simulink model "rusticone"  (R2018b)
settings: Solver=VariableStepAuto  StartTime=0.0  StopTime=10.0  RelTol=1e-3
libraries: simulink_extras x1, simulink x1
settings Model: Creator=Edoardo  LastModifiedBy=Edoardo

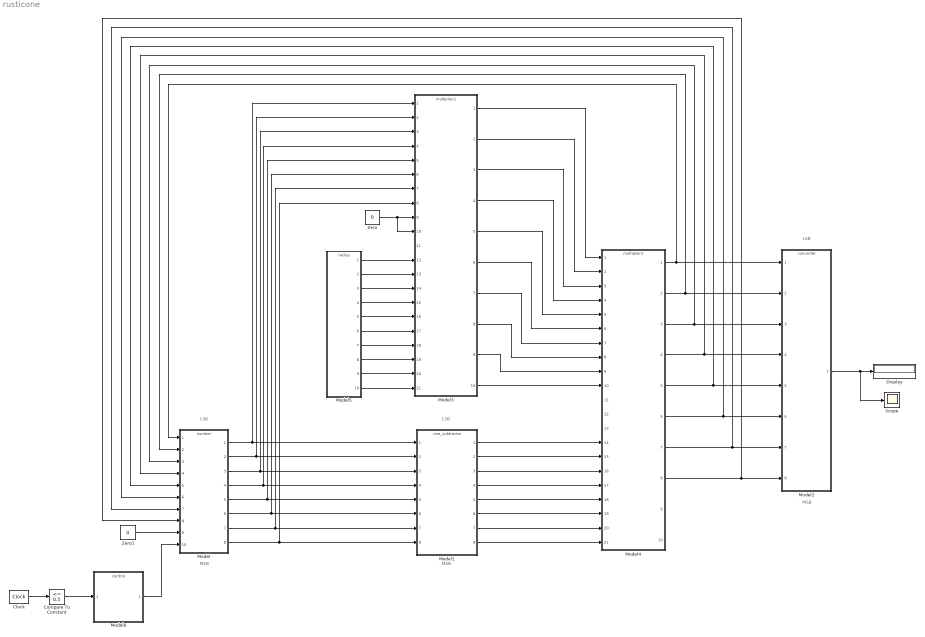
== system rusticone ==
  note: LSB
  note: LSB
  note: MSB
  note: LSB
  note: MSB
  note: MSB
  Clock : simulink_extras/Flip Flops/Clock  period=2
  Compare To Constant : simulink/Logic and Bit Operations/Compare To Constant  relop=<=  const=0.5  OutDataTypeStr=boolean  ZeroCross=off
  Display : Display
  Model : ModelReference  ModelNameDialog=number  SimulationMode=Normal  ModelReferenceVersion=1.14
  Model1 : ModelReference  ModelNameDialog=one_subtractor  SimulationMode=Normal  ModelReferenceVersion=1.7
  Model2 : ModelReference  ModelNameDialog=converter  SimulationMode=Normal  ModelReferenceVersion=1.8
  Model3 : ModelReference  ModelNameDialog=multiplier2.slx  SimulationMode=Normal  ModelReferenceVersion=1.12
  Model4 : ModelReference  ModelNameDialog=multiplier2.slx  SimulationMode=Normal  ModelReferenceVersion=1.12
  Model5 : ModelReference  ModelNameDialog=radius  SimulationMode=Normal  ModelReferenceVersion=1.3
  Model6 : ModelReference  ModelNameDialog=control  SimulationMode=Normal  ModelReferenceVersion=1.1
  Scope : Scope
  Zero : Constant  Value=0  OutDataTypeStr=Inherit: Inherit via back propagation
  Zero1 : Constant  Value=0  OutDataTypeStr=Inherit: Inherit via back propagation
  wires:
  Model2/1 -> Scope/1, Display/1
  Model/1 -> Model3/1, Model1/1
  Model/6 -> Model3/6, Model1/6
  Model/7 -> Model3/7, Model1/7
  Model/4 -> Model1/4, Model3/4
  Model/8 -> Model3/8, Model1/8
  Model/2 -> Model3/2, Model1/2
  Model/5 -> Model3/5, Model1/5
  Model/3 -> Model3/3, Model1/3
  Model3/1 -> Model4/1
  Model3/2 -> Model4/2
  Model3/3 -> Model4/3
  Model3/4 -> Model4/4
  Model3/5 -> Model4/5
  Model3/6 -> Model4/6
  Model3/7 -> Model4/7
  Model3/8 -> Model4/8
  Model3/9 -> Model4/9
  Model3/10 -> Model4/10
  Model1/1 -> Model4/14
  Model1/2 -> Model4/15
  Model1/3 -> Model4/16
  Model1/4 -> Model4/17
  Model1/5 -> Model4/18
  Model1/6 -> Model4/19
  Model1/7 -> Model4/20
  Model1/8 -> Model4/21
  Zero/1 -> Model3/10, Model3/9
  Model4/1 -> Model2/1, Model/1
  Model4/2 -> Model2/2, Model/2
  Model4/3 -> Model2/3, Model/3
  Model4/4 -> Model/4, Model2/4
  Model4/5 -> Model2/5, Model/5
  Model4/6 -> Model2/6, Model/6
  Model4/7 -> Model2/7, Model/7
  Model4/8 -> Model/8, Model2/8
  Model5/1 -> Model3/12
  Model5/2 -> Model3/13
  Model5/3 -> Model3/14
  Model5/4 -> Model3/15
  Model5/5 -> Model3/16
  Model5/6 -> Model3/17
  Model5/7 -> Model3/18
  Model5/8 -> Model3/19
  Model5/9 -> Model3/20
  Model5/10 -> Model3/21
  Clock/1 -> Compare To Constant/1
  Model6/1 -> Model/10
  Zero1/1 -> Model/9
  Compare To Constant/1 -> Model6/1
